simulink model "exakt_siso"  (Simulink 2.20)
settings: Solver=ode45  StartTime=0.0  StopTime=20.0  MaxStep=0.1  RelTol=1e-3  AbsTol=1e-6
libraries: NelinSys x4
CloseFcn:
  | ;slview('closediagram',bdroot);
settings Model: ConsistencyChecking=off  RTWPlaceOutputsASAP=off

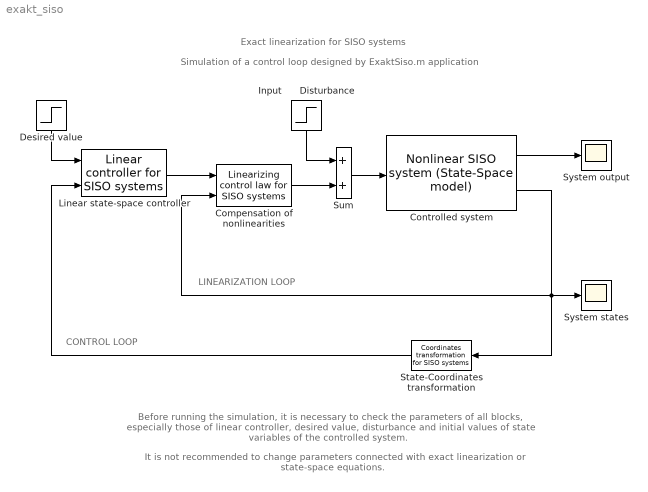
== system exakt_siso ==
  note: LINEARIZATION LOOP
  note: CONTROL LOOP
  note: Exact linearization for SISO systems
  note: Simulation of a control loop designed by ExaktSiso.m application
  note: Before running the simulation, it is necessary to check the parameters of all blocks, especially those
      | of linear controller, desired value, disturbance and initial values of state variables of the controlled system.
  note: It is not recommended to change parameters connected with exact linearization or state-space equations.
  Compensation of nonlinearities : NelinSys/Nonlinear Systems Synthesis/Exact Linearization Blocks/Linearizing control law for SISO systems  n=n  vzorecP=u
  Controlled system : NelinSys/Nonlinear Systems Synthesis/Nonlinear SISO system (State-Space model)  n=n  Fp=F  Gp=G  Hp=H  pp=[0.1; 0.01]
  Desired value : Step  Orientation=down  Time=5  Before=2  After=10
  Input      Disturbance : Step  Orientation=down  Time=15  Before=0  After=1
  Linear state-space controller : NelinSys/Nonlinear Systems Synthesis/Exact Linearization Blocks/Linear controller for SISO systems  r=r  kor=[-2 -2 -6]  integ=on
  State-Coordinates transformation : NelinSys/Nonlinear Systems Synthesis/Exact Linearization Blocks/Coordinates transformation for SISO systems  Orientation=left  n=n  r=r  Zp=qx
  Sum : Sum  Inputs=++
  System output : Scope
      settings: TickLabels=on  TimeRange=auto  YMin=-5  YMax=5  SaveToWorkspace=off  SaveName=ScopeData
  System states : Scope
      settings: TickLabels=on  TimeRange=auto  YMin=-5  YMax=5  SaveToWorkspace=off  SaveName=ScopeData
  wires:
  Linear state-space controller/1 -> Compensation of nonlinearities/1
  Compensation of nonlinearities/1 -> Sum/2
  Sum/1 -> Controlled system/1
  Controlled system/2 -> State-Coordinates transformation/1, Compensation of nonlinearities/2, System states/1
  Controlled system/1 -> System output/1
  Input      Disturbance/1 -> Sum/1
  State-Coordinates transformation/1 -> Linear state-space controller/2
  Desired value/1 -> Linear state-space controller/1
